simulink model "PMSM_motorModel"  (R2024b)
settings: Solver=VariableStepAuto  StartTime=0.0  StopTime=10.0  RelTol=1e-3
undefined symbols (not defined in the file or in its folder): mot
settings Model: Creator=giulio  LastModifiedBy=giulio

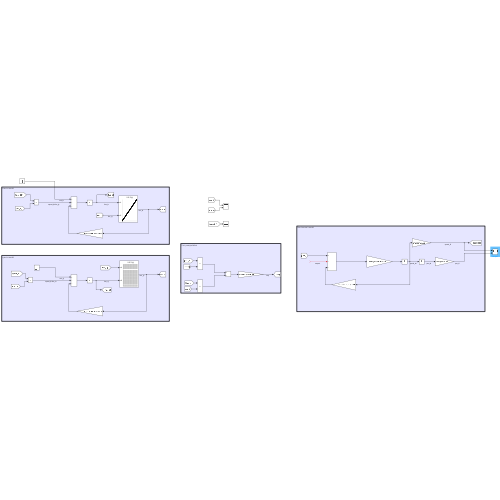
[thumbnail: Simulink's stored preview of the top-level diagram]
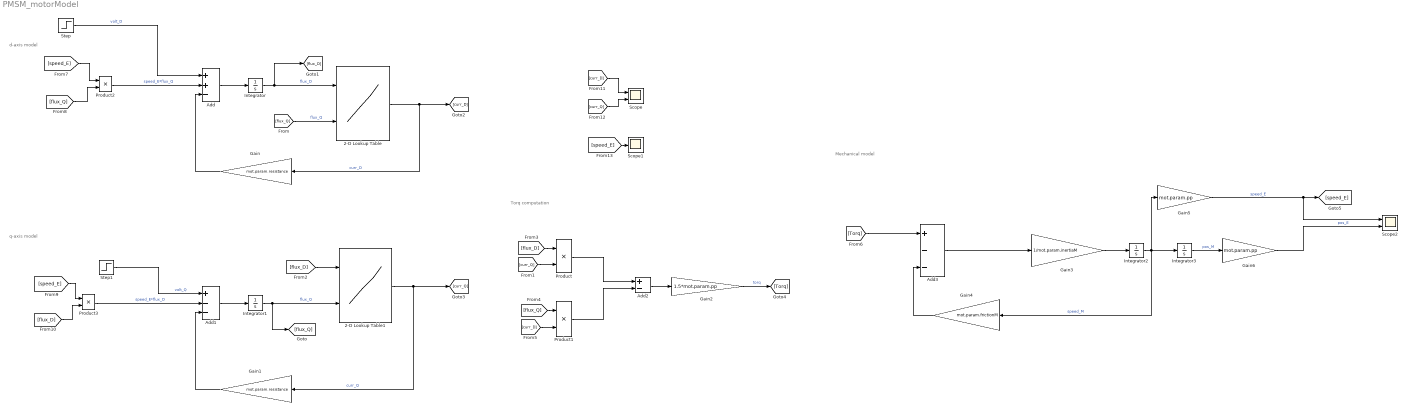
== system PMSM_motorModel ==
  note: Mechanical model
  note: Torq computation
  note: d-axis model
  note: q-axis model
  2-D Lookup Table : Lookup_n-D  BreakpointsForDimension1=mot.maps.fluxVec_D  BreakpointsForDimension2=mot.maps.fluxVec_Q  Table=mot.maps.currMap_D'  InternalRulePriority=Speed  RndMeth=Simplest
      settings: InputPortMap=u0,u1
  2-D Lookup Table1 : Lookup_n-D  BreakpointsForDimension1=mot.maps.fluxVec_D  BreakpointsForDimension2=mot.maps.fluxVec_Q  Table=mot.maps.currMap_Q'  InternalRulePriority=Speed  RndMeth=Simplest
      settings: InputPortMap=u0,u1
  Add : Sum  Inputs=++-
  Add1 : Sum  Inputs=+--
  Add2 : Sum  Inputs=+-
  Add3 : Sum  Inputs=+--
  Gain : Gain  Gain=mot.param.resistance
  Gain1 : Gain  Gain=mot.param.resistance
  Gain2 : Gain  Gain=1.5*mot.param.pp
  Gain3 : Gain  Gain=1/mot.param.inertiaM
  Gain4 : Gain  Gain=mot.param.frictionM
  Gain5 : Gain  Gain=mot.param.pp
  Gain6 : Gain  Gain=mot.param.pp
  Integrator : Integrator  InitialCondition=mot.param.fluxPM
  Integrator1 : Integrator
  Integrator2 : Integrator
  Integrator3 : Integrator
  Product{,1..3} (4 alike) : Product
  Scope : Scope  NumInputPorts=2
  Scope1 : Scope
  Scope2 : Scope  NumInputPorts=2
  Step : Step  SampleTime=0
  Step1 : Step  Time=2  SampleTime=0
  wires:
  Integrator/1 -> [flux_D], 2-D Lookup Table/1  "flux_D"
  [flux_Q] -> 2-D Lookup Table/2  "flux_Q"
  Add/1 -> Integrator/1
  Step/1 -> Add/1  "volt_D"
  Product2/1 -> Add/2  "speed_E*flux_Q"
  2-D Lookup Table/1 -> [curr_D], Gain/1  "curr_D"
  Gain/1 -> Add/3
  2-D Lookup Table1/1 -> [curr_Q], Gain1/1  "curr_Q"
  Gain1/1 -> Add1/3
  Step1/1 -> Add1/1  "volt_Q"
  Integrator1/1 -> [flux_Q], 2-D Lookup Table1/2  "flux_Q"
  Add1/1 -> Integrator1/1
  Product3/1 -> Add1/2  "speed_E*flux_D"
  [flux_D] -> 2-D Lookup Table1/1
  [flux_D] -> Product/1
  [curr_Q] -> Product/2
  [flux_Q] -> Product1/1
  [curr_D] -> Product1/2
  Product/1 -> Add2/1
  Product1/1 -> Add2/2
  Add2/1 -> Gain2/1
  Gain2/1 -> [Torq]  "torq"
  Integrator2/1 -> Gain5/1, Gain4/1, Integrator3/1  "speed_M"
  Integrator3/1 -> Gain6/1  "pos_M"
  Gain3/1 -> Integrator2/1
  [Torq] -> Add3/1
  Add3/1 -> Gain3/1
  ? -> Add3/2  "torqueL"
  Gain4/1 -> Add3/3
  Gain5/1 -> Scope2/1, [speed_E]  "speed_E"
  Gain6/1 -> Scope2/2  "pos_E"
  [flux_Q] -> Product2/2
  [speed_E] -> Product2/1
  [speed_E] -> Product3/1
  [flux_D] -> Product3/2
  [curr_D] -> Scope/1
  [curr_Q] -> Scope/2
  [speed_E] -> Scope1/1
